simulink model "L0607"  (Simulink 9.1)
settings: Solver=VariableStepDiscrete  StartTime=0.0  StopTime=10.0  MaxStep=0.01  RelTol=1e-3
InitFcn:
  | data
values from neighbouring files (symbols this model uses):
  Alpha = 65    [data.m]
  g = 9.81    [data.m]
  Vx0 = 5    [data.m]
  Vy0 = 16    [data.m]
  x0 = 1    [data.m]
  y0 = 5    [data.m]
libraries: simulink x1
settings Model: Creator=Asus  LastModifiedBy=Asus
settings DataIOCC: SaveFormat=Dataset
settings OptimizationCC: LifeSpan=auto
settings DebuggingCC: UnderspecifiedInitializationDetection=Simplified  MergeDetectMultiDrivingBlocksExec=error  SFUnexpectedBacktrackingDiag=error  SFNoUnconditionalDefaultTransitionDiag=error  SFExecutionAtInitializationDiag=warning
settings HardwareCC: ProdBitPerPointer=64  ProdBitPerSizeT=64  ProdBitPerPtrDiffT=64  ProdLargestAtomicFloat=Float  ProdIntDivRoundTo=Zero  ProdEndianess=LittleEndian  ProdWordSize=64  ProdHWDeviceType=Intel->x86-64 (Windows64)
settings ModelReferenceCC: PropagateSignalLabelsOutOfModel=on
settings CodeAppCC: StateflowObjectComments=off
settings GRTTargetCC: TargetLangStandard=C99 (ISO)  CombineOutputUpdateFcns=on  GRTInterface=off
settings ConfigComp: CovMetricSettings=dwe  CovHtmlReporting=off  CovSaveCumulativeToWorkspaceVar=off  CovSaveSingleToWorkspaceVar=off  CovExternalEMLEnable=on

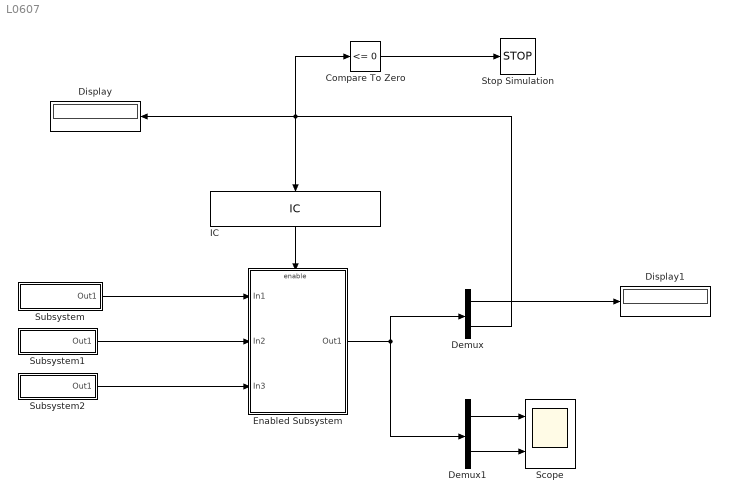
== system L0607 ==
  Compare To Zero : simulink/Logic and Bit Operations/Compare To Zero  relop=<=  OutDataTypeStr=boolean
  Demux : Demux  Outputs=2
  Demux1 : Demux  Outputs=2
  Display : Display
  Display1 : Display
  Enabled Subsystem : Subsystem  TreatAsAtomicUnit=on
  IC : InitialCondition  Value=[y0 | sqrt(Vx0^2+Vy0^2)]
  Scope : Scope  NumInputPorts=2
  Stop Simulation : Stop
  Subsystem : Subsystem
  Subsystem1 : Subsystem
  Subsystem2 : Subsystem
  wires:
  Compare To Zero/1 -> Stop Simulation/1
  Demux/2 -> Compare To Zero/1, Display/1, IC/1
  Enabled Subsystem/1(Out1) -> Demux1/1, Demux/1
  Subsystem/1(Out1) -> Enabled Subsystem/1(In1)
  IC/1 -> Enabled Subsystem/Enable
  Subsystem1/1(Out1) -> Enabled Subsystem/2(In2)
  Subsystem2/1(Out1) -> Enabled Subsystem/3(In3)
  Demux1/1 -> Scope/1
  Demux1/2 -> Scope/2
  Demux/1 -> Display1/1

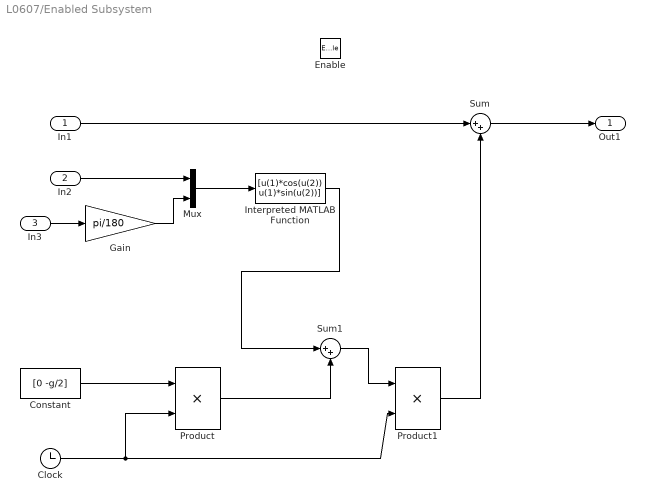
== system L0607/Enabled Subsystem ==
  In1 : Inport
  In2 : Inport  Port=2
  In3 : Inport  Port=3
  Enable : EnablePort
  Clock : Clock
  Constant : Constant  Value=[0 -g/2]
  Gain : Gain  Gain=pi/180
  Interpreted MATLAB Function : MATLABFcn  MATLABFcn=[u(1)*cos(u(2)) u(1)*sin(u(2))]
  Mux : Mux  Inputs=2
  Product : Product
  Product1 : Product
  Sum : Sum  Inputs=|++
  Sum1 : Sum  Inputs=|++
  Out1 : Outport
  wires:
  Constant/1 -> Product/1
  Clock/1 -> Product/2, Product1/2
  In1/1 -> Sum/1
  Product/1 -> Sum1/2
  Sum1/1 -> Product1/1
  Product1/1 -> Sum/2
  Sum/1 -> Out1/1
  In3/1 -> Gain/1
  In2/1 -> Mux/1
  Gain/1 -> Mux/2
  Mux/1 -> Interpreted MATLAB Function/1
  Interpreted MATLAB Function/1 -> Sum1/1

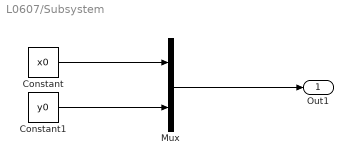
== system L0607/Subsystem ==
  Constant : Constant  Value=x0
  Constant1 : Constant  Value=y0
  Mux : Mux  Inputs=2
  Out1 : Outport
  wires:
  Constant/1 -> Mux/1
  Constant1/1 -> Mux/2
  Mux/1 -> Out1/1

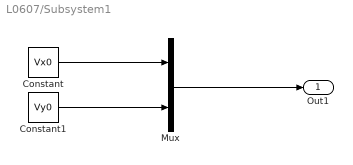
== system L0607/Subsystem1 ==
  Constant : Constant  Value=Vx0
  Constant1 : Constant  Value=Vy0
  Mux : Mux  Inputs=2
  Out1 : Outport
  wires:
  Constant/1 -> Mux/1
  Constant1/1 -> Mux/2
  Mux/1 -> Out1/1

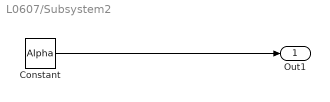
== system L0607/Subsystem2 ==
  Constant : Constant  Value=Alpha
  Out1 : Outport
  wires:
  Constant/1 -> Out1/1
